simulink model "SMC_for_Mass_Spring_Damper_System_With_Disturbance"  (Simulink 9.3)
settings: Solver=FixedStepAuto  StartTime=0.0  StopTime=10  FixedStep=0.01  RelTol=1e-3
settings Model: LogicAnalyzerSignalOrdering=4583f6d2-b4a9-433d-9afe-2cb38677ff06,7c2acc27-c43a-428c-972b-34ad91a8f535,2fe628d0-ec7f-45c5-b406-8622b80bae60,ebdcd677-7f0e-4fbb-9a40-b8d4573ad7d3  Creator=User2  LastModifiedBy=User2
settings DataIOCC: SaveFormat=Dataset  SignalLoggingSaveFormat=Dataset  ReturnWorkspaceOutputs=on
settings OptimizationCC: LifeSpan=auto
settings DebuggingCC: UnderspecifiedInitializationDetection=Simplified  MergeDetectMultiDrivingBlocksExec=error  FcnCallInpInsideContextMsg=error  SFUnexpectedBacktrackingDiag=error  SFNoUnconditionalDefaultTransitionDiag=error  SFExecutionAtInitializationDiag=warning  ArithmeticOperatorsInVariantConditions=error
settings HardwareCC: ProdBitPerPointer=64  ProdBitPerSizeT=64  ProdBitPerPtrDiffT=64  ProdLargestAtomicFloat=Float  ProdIntDivRoundTo=Zero  ProdEndianess=LittleEndian  ProdWordSize=64  ProdHWDeviceType=Intel->x86-64 (Windows64)
settings ModelReferenceCC: PropagateSignalLabelsOutOfModel=on
settings SFSimCC: SimUseLocalCustomCode=on
settings RTWCC: RTWUseLocalCustomCode=on
settings CodeAppCC: StateflowObjectComments=off
settings GRTTargetCC: TargetLangStandard=C99 (ISO)  CombineOutputUpdateFcns=on  GRTInterface=off
settings ConfigComp: CovMetricSettings=dwe  CovHtmlReporting=off  CovSaveCumulativeToWorkspaceVar=off  CovSaveSingleToWorkspaceVar=off  CovExternalEMLEnable=on

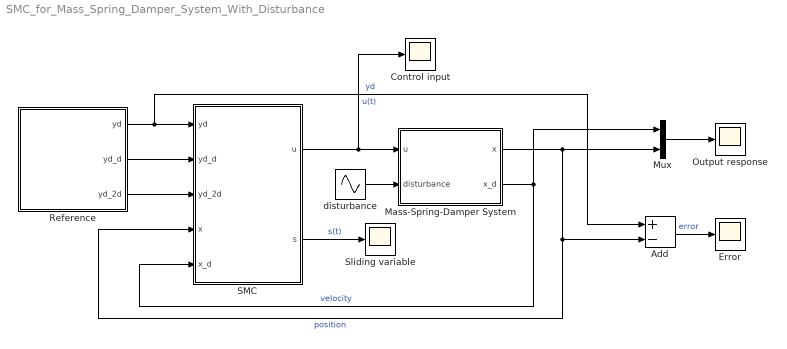
== system SMC_for_Mass_Spring_Damper_System_With_Disturbance ==
  Add : Sum  Inputs=+-
  Control input : Scope
  Error : Scope
  Mass-Spring-Damper System : Subsystem
  Mux : Mux  Inputs=2
  Output response : Scope
  Reference : Subsystem
  SMC : MATLAB Function  TreatAsAtomicUnit=on
  Sliding variable : Scope
  disturbance : Sin  Amplitude=0.5  SampleTime=0
  wires:
  SMC/1(u) -> Control input/1, Mass-Spring-Damper System/1(u)  "u(t)"
  Reference/1(yd) -> SMC/1(yd), Add/1  "yd"
  Reference/2(yd_d) -> SMC/2(yd_d)
  Reference/3(yd_2d) -> SMC/3(yd_2d)
  Mux/1 -> Output response/1
  Add/1 -> Error/1  "error"
  SMC/2(s) -> Sliding variable/1  "s(t)"
  Mass-Spring-Damper System/1(x) -> Mux/2, SMC/4(x), Add/2  "position"
  Mass-Spring-Damper System/2(x_d) -> Mux/1, SMC/5(x_d)  "velocity"
  disturbance/1 -> Mass-Spring-Damper System/2(disturbance)

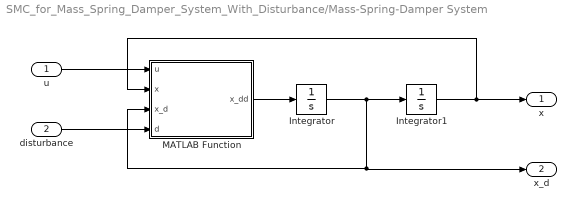
== system SMC_for_Mass_Spring_Damper_System_With_Disturbance/Mass-Spring-Damper System ==
  u : Inport
  disturbance : Inport  Port=2
  Integrator : Integrator
  Integrator1 : Integrator  InitialCondition=1
  MATLAB Function : MATLAB Function  TreatAsAtomicUnit=on
  x : Outport
  x_d : Outport  Port=2
  wires:
  u/1 -> MATLAB Function/1(u)
  MATLAB Function/1(x_dd) -> Integrator/1
  Integrator/1 -> Integrator1/1, x_d/1, MATLAB Function/3(x_d)
  Integrator1/1 -> x/1, MATLAB Function/2(x)
  disturbance/1 -> MATLAB Function/4(d)

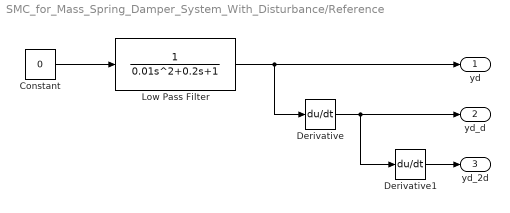
== system SMC_for_Mass_Spring_Damper_System_With_Disturbance/Reference ==
  Constant : Constant  Value=0
  Derivative : Derivative
  Derivative1 : Derivative
  Low Pass Filter : TransferFcn  Denominator=[0.01 0.2 1]
  yd : Outport
  yd_d : Outport  Port=2
  yd_2d : Outport  Port=3
  wires:
  Constant/1 -> Low Pass Filter/1
  Low Pass Filter/1 -> Derivative/1, yd/1
  Derivative/1 -> Derivative1/1, yd_d/1
  Derivative1/1 -> yd_2d/1

== matlab function Mass-Spring-Damper System/MATLAB Function ==
  data: u input double; x input double; x_dd output double; x_d input double; d input double
function x_dd = Dynamic(u, x, x_d, d)
%% Declaration
D=0.1; % damping coefficient-Ns/m
M=1; % Mass-kg
K=1; % Spring constant-N/m

f=-(D*x_d+K*x)/M; %  inherent forces of the damper and spring acting on the mass
gg=1/M; % signifies the influence of the control force F on the mass, normalized by its magnitude

%% Simulation
x_dd=f+gg*u+d;

== matlab function SMC ==
  data: yd input double; yd_d input double; yd_2d input double; u output double; x input double; x_d input double; s output double
function [u,s]= SMC(yd, yd_d, yd_2d, x, x_d)
%% Declaration
D=0.1; % damping coefficient-Ns/m
M=1; % Mass-kg
K=1; % Spring constant-N/m

k=3;
eta=0.1;
lamda=5;
d=0.6;

f=-(D*x_d+K*x)/M; %  inherent forces of the damper and spring acting on the mass
gg=1/M; % signifies the influence of the control force F on the mass, normalized by its magnitude

e=yd-x;
e_d=yd_d-x_d;
s=e_d+lamda*e;

%% Control output
u=(1/gg)*(yd_2d+lamda*e_d-f+k*s+eta*sign(s)+d*sign(s));
